simulink model "sampleModel371"  (R2021b)
settings: Solver=VariableStepAuto  StartTime=0.0  StopTime=10.0  RelTol=1e-3
undefined symbols (not defined in the file or in its folder): DiscIntNeverNeededParam, Newton, Raphson
libraries: simulink x16, slpidlib x1
settings Model: Creator=user  LastModifiedBy=user

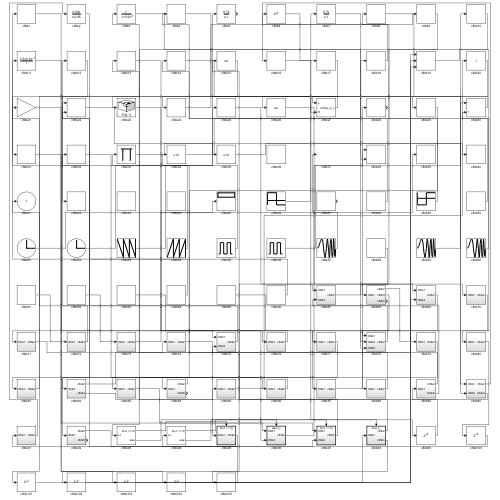
[thumbnail: Simulink's stored preview of the top-level diagram]
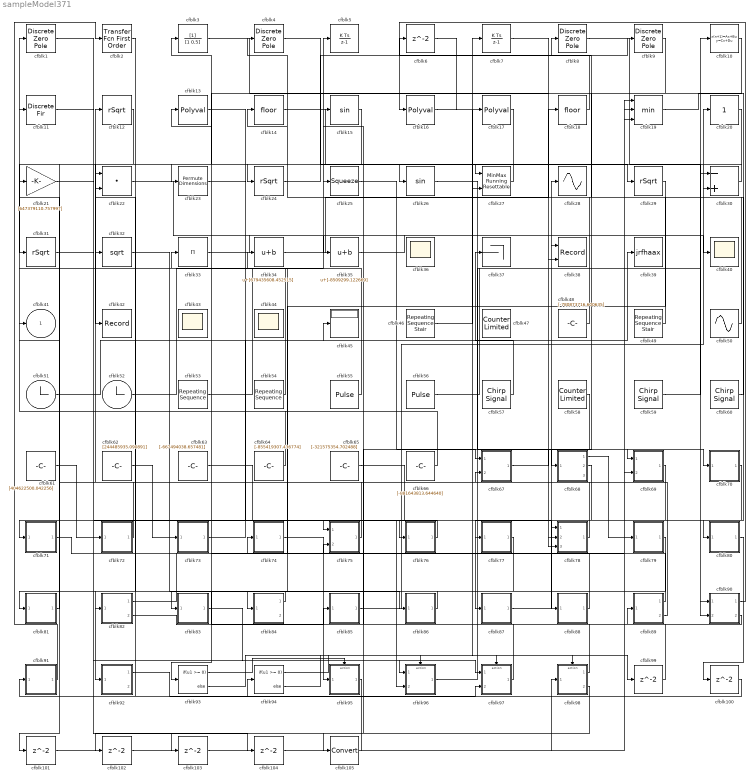
== system sampleModel371 ==
  cfblk{1,4,8..9} (4 alike) : DiscreteZeroPole  Poles=[0 0.5]  Gain=1
  cfblk10 : DiscreteStateSpace
  cfblk{6,99..104} (7 alike) : Delay  SampleTime=1
  cfblk105 : DataTypeConversion
  cfblk11 : DiscreteFir  SampleTime=1
  cfblk{12,24,29,31} (4 alike) : Sqrt  Operator=rSqrt  AlgorithmType=Newton-Raphson  SaturateOnIntegerOverflow=on
  cfblk13 : Polyval  Coefs=[ +2.081618890e-019, -1.441693666e-014, +4.719686976e-010, -8.536869453e-006, +1.621573104e-001, -8.087801117e+001 ]
  cfblk14 : Rounding
  cfblk15 : Trigonometry
  cfblk16 : Polyval  Coefs=[ +2.081618890e-019, -1.441693666e-014, +4.719686976e-010, -8.536869453e-006, +1.621573104e-001, -8.087801117e+001 ]
  cfblk17 : Polyval  Coefs=[ +2.081618890e-019, -1.441693666e-014, +4.719686976e-010, -8.536869453e-006, +1.621573104e-001, -8.087801117e+001 ]
  cfblk18 : Rounding
  cfblk19 : MinMax  Inputs=3
  cfblk2 : simulink/Discrete/Transfer Fcn First Order  PoleZ=0.95  ICPrevOutput=0.0  DoSatur=off
  cfblk20 : simulink/Math Operations/Slider Gain  gain=1  low=0  high=2
  cfblk21 : Gain  Gain=[647379110.757997]
  cfblk22 : DotProduct  InputSameDT=on  OutDataTypeStr=Inherit: Inherit via internal rule
  cfblk23 : PermuteDimensions
  cfblk25 : Squeeze
  cfblk26 : Trigonometry
  cfblk27 : simulink/Math Operations/MinMax Running Resettable  Function=min  vinit=0.0
  cfblk28 : Sin  TimeSource=Use external signal  SampleTime=0
  cfblk3 : DiscreteFilter  SampleTime=1
  cfblk30 : Sum  Inputs=-+
  cfblk32 : Sqrt  SaturateOnIntegerOverflow=on
  cfblk33 : Product  Inputs=*
  cfblk34 : Bias  Bias=[679435608.452515]
  cfblk35 : Bias  Bias=[-8509299.122669]
  cfblk{36,40,43..44} (4 alike) : Scope
      cfblk36 settings: Floating=on
      cfblk43 settings: Floating=on
      cfblk44 settings: Floating=on
  cfblk37 : Terminator
  cfblk38 : Record  FileSettingsInternal="{\"entries\":[{\"content\":{\"excelSettings\":{\"content\":{},\"type\":\"Streamout.ExcelSettings\"}},\"type\":\"Streamout.FileSettingStorage\",\"uuid\":\"9fc04052-8b8e-4725-86d2-7cf5f812b2a1\"}],\"packageUris\":[\"http://schema.mathworks.com/mf0/streamout_blocks/R2020a\"],\"version\":\"1.0\"}"  Layout=[1 1]  SignalsInternal="{\"entries\":[{\"content\":{\"signals\":[{\"content\":{\"blockPath\":[\"sampleModel371/cfblk38\"],\"channel\":[],\"dimensions\":[1],\"domain\":\"sampleModel371/cfblk38\",\"lineColor\":\"#a2142f\",\"plots\":[1],\"port\":1,\"sid\":[\"\"],\"signalID\":15418,\"signalName\":\"cfblk96\"},\"type\":\"RecordBlkView.Signal\",\"uuid\":\"3d61ea52-26a8-4207-9b7d-ce4d298dc0bd\"},{\"content\":{\"blockPath\":[\"sampleModel371/cfblk38\"],\"channel\":[],\"dimensions\":[1],\"domain\":\"sampleModel371/cfblk38\",\"lineColor\":\"#139fff\",\"plots\":[1],\"port\":2,\"sid\":[\"\"],\"signalID\":15422,\"signalName\":\"cfblk3\"},\"type\":\"RecordBlkView.Signal\",\"uuid\":\"41d0d82b-847e-4e7e-9938-72f6bd31de9c\"}]},\"type\":\"RecordBlkView.InputSignals\",\"uuid\":\"d21ca9dd-40f7-4d18-b4d9-355bbf76461b\"}],\"packageUris\":[\"http://schema.mathworks.com/mf0/streamout_blocks/R2020a\"],\"version\":\"1.0\"}"  VisualizationBindings="{\"xyplotplugin\":{\"info\":[{\"series\":[{\"bindingParametersList\":[{\"parameter\":\"X-Axis\",\"signalID\":15418,\"signalName\":\"cfblk96\"},{\"parameter\":\"Y-Axis\",\"signalID\":15422,\"signalName\":\"cfblk3\"}],\"seriesID\":59305}],\"subplotID\":1}]}}"  CompatibilityTag=XY
  cfblk39 : ToWorkspace  VariableName=jrfhaax  SaveFormat=Timeseries  SampleTime=-1
  cfblk42 : Record  FileSettingsInternal="{\"entries\":[{\"content\":{\"excelSettings\":{\"content\":{},\"type\":\"Streamout.ExcelSettings\"}},\"type\":\"Streamout.FileSettingStorage\",\"uuid\":\"b9a56b8f-e8fc-4666-a556-652c0deea9d6\"}],\"packageUris\":[\"http://schema.mathworks.com/mf0/streamout_blocks/R2020a\"],\"version\":\"1.0\"}"  SignalsInternal="{\"entries\":[{\"content\":{\"signals\":[{\"content\":{\"blockPath\":[\"sampleModel371/cfblk42\"],\"channel\":[],\"dimensions\":[1],\"domain\":\"sampleModel371/cfblk42\",\"lineColor\":\"#0072bd\",\"plots\":[1],\"port\":1,\"sid\":[\"\"],\"signalID\":15426,\"signalName\":\"cfblk12\"},\"type\":\"RecordBlkView.Signal\",\"uuid\":\"61be2cdd-bcd1-4740-b751-c89f055e617a\"}]},\"type\":\"RecordBlkView.InputSignals\",\"uuid\":\"9fe64509-3397-4dbe-9be9-cbf438e67b07\"}],\"packageUris\":[\"http://schema.mathworks.com/mf0/streamout_blocks/R2020a\"],\"version\":\"1.0\"}"  VisualizationBindings="{\"sparklinesplugin\":{\"info\":[{\"bindingParametersList\":[],\"subplotID\":1}]}}"
  cfblk45 : Display
  cfblk46 : simulink/Sources/Repeating Sequence Stair  OutValues=[875396539.416185, -474636717.858967]  tsamp=-1  OutMin=[]  OutMax=[]  OutDataTypeStr=double  OutputDataTypeScalingMode=double  OutDataType=fixdt(0,8)  ConRadixGroup=Best Precision: Vector-wise  OutScaling=2^-12
  cfblk47 : simulink/Sources/Counter Limited  uplimit=[503.000000]  tsamp=-1
  cfblk48 : Constant  Value=[-780873716.600635]  SampleTime=1
  cfblk49 : simulink/Sources/Repeating Sequence Stair  OutValues=[-638428813.350056, 591562095.048275]  tsamp=-1  OutMin=[]  OutMax=[]  OutDataTypeStr=double  OutputDataTypeScalingMode=double  OutDataType=fixdt(0,8)  ConRadixGroup=Best Precision: Vector-wise  OutScaling=2^-12
  cfblk5 : DiscreteIntegrator  ICPrevOutput=DiscIntNeverNeededParam  ICPrevScaledInput=DiscIntNeverNeededParam
  cfblk50 : Sin  Amplitude=[814277309.759991]  Bias=[541474944.272401]  SampleTime=0
  cfblk51 : Clock
  cfblk52 : Clock
  cfblk53 : simulink/Sources/Repeating Sequence  rep_seq_t=[0 2]  rep_seq_y=[845598194.254567, 45370993.914203]
  cfblk54 : simulink/Sources/Repeating Sequence  rep_seq_t=[0 2]  rep_seq_y=[-622327897.536918, 514712392.669646]
  cfblk55 : DiscretePulseGenerator  PulseType=Time based  Amplitude=[944860863.611499]  Period=[65183913.372249]  PulseWidth=5  PhaseDelay=[8.000000]
  cfblk56 : DiscretePulseGenerator  PulseType=Time based  Amplitude=[-618955552.202892]  Period=[96517376.948850]  PulseWidth=5  PhaseDelay=[6.000000]
  cfblk57 : simulink/Sources/Chirp Signal  f1=[-190410484.852389]  T=[-195836475.301159]  f2=[603076761.049047]
  cfblk58 : simulink/Sources/Counter Limited  uplimit=[276.000000]  tsamp=-1
  cfblk59 : simulink/Sources/Chirp Signal  f1=[606511793.008932]  T=[320109653.210944]  f2=[959584980.441346]
  cfblk60 : simulink/Sources/Chirp Signal  f1=[-875766691.668898]  T=[126991163.871729]  f2=[-767987395.473026]
  cfblk61 : Constant  Value=[404622500.042256]  SampleTime=1
  cfblk62 : Constant  Value=[244485935.090891]  SampleTime=1
  cfblk63 : Constant  Value=[-667494038.657481]  SampleTime=1
  cfblk64 : Constant  Value=[-855419307.436774]  SampleTime=1
  cfblk65 : Constant  Value=[-321575354.702488]  SampleTime=1
  cfblk66 : Constant  Value=[-881643813.644640]  SampleTime=1
  cfblk67 : Subsystem
  cfblk68 : Subsystem
  cfblk69 : Subsystem
  cfblk7 : DiscreteIntegrator  ICPrevOutput=DiscIntNeverNeededParam  ICPrevScaledInput=DiscIntNeverNeededParam
  cfblk70 : Subsystem
  cfblk71 : Subsystem
  cfblk72 : Subsystem
  cfblk73 : Subsystem
  cfblk74 : Subsystem
  cfblk75 : Subsystem
  cfblk76 : Subsystem
  cfblk77 : Subsystem
  cfblk78 : Subsystem
  cfblk79 : Subsystem
  cfblk80 : Subsystem
  cfblk81 : Subsystem
  cfblk82 : Subsystem
  cfblk83 : Subsystem
  cfblk84 : Subsystem
  cfblk85 : Subsystem
  cfblk86 : Subsystem
  cfblk87 : Subsystem
  cfblk88 : Subsystem
  cfblk89 : Subsystem
  cfblk90 : Subsystem
  cfblk91 : Subsystem
  cfblk92 : Subsystem
  cfblk93 : If  IfExpression=u1 >= 0  SampleTime=1
  cfblk94 : If  IfExpression=u1 >= 0  SampleTime=1
  cfblk95 : Subsystem  TreatAsAtomicUnit=on
  cfblk96 : Subsystem  TreatAsAtomicUnit=on
  cfblk97 : Subsystem  TreatAsAtomicUnit=on
  cfblk98 : Subsystem  TreatAsAtomicUnit=on
  cfblk41 : Outport
  wires:
  cfblk51/1 -> cfblk39/1
  cfblk61/1 -> cfblk72/1(cfblk1)
  cfblk85/1(cfblk2) -> cfblk20/1
  cfblk62/1 -> cfblk73/1(cfblk1)
  cfblk76/1(cfblk2) -> cfblk71/1(cfblk1)
  cfblk87/1(cfblk2) -> cfblk28/1
  cfblk71/1(cfblk2) -> cfblk74/1(cfblk1)
  cfblk96/1(cfblk2) -> cfblk38/1
  cfblk49/1 -> cfblk8/1
  cfblk64/1 -> cfblk1/1
  cfblk29/1 -> cfblk84/1(cfblk1)
  cfblk72/1(cfblk2) -> cfblk12/1
  cfblk52/1 -> cfblk5/1
  cfblk65/1 -> cfblk87/1(cfblk1)
  cfblk35/1 -> cfblk40/1
  cfblk19/1 -> cfblk80/1(cfblk1)
  cfblk81/1(cfblk2) -> cfblk41/1
  cfblk79/1(cfblk2) -> cfblk92/1(cfblk1)
  cfblk12/1 -> cfblk42/1
  cfblk90/1(cfblk2) -> cfblk16/1
  cfblk9/1 -> cfblk68/1(cfblk1)
  cfblk59/1 -> cfblk10/1
  cfblk86/1(cfblk2) -> cfblk81/1(cfblk1)
  cfblk30/1 -> cfblk26/1
  cfblk26/1 -> cfblk70/1(cfblk1)
  cfblk83/1(cfblk2) -> cfblk96/1(cfblk1)
  cfblk74/1(cfblk2) -> cfblk95/1(cfblk1)
  cfblk56/1 -> cfblk30/1
  cfblk55/1 -> cfblk11/1
  cfblk4/1 -> cfblk29/1
  cfblk97/1(cfblk2) -> cfblk13/1
  cfblk54/1 -> cfblk3/1
  cfblk60/1 -> cfblk30/2
  cfblk20/1 -> cfblk31/1
  cfblk68/1(cfblk2) -> cfblk79/1(cfblk1)
  cfblk27/1 -> cfblk24/1
  cfblk53/1 -> cfblk25/1
  cfblk73/1(cfblk2) -> cfblk45/1
  cfblk48/1 -> cfblk14/1
  cfblk34/1 -> cfblk18/1
  cfblk75/1(cfblk2) -> cfblk22/1
  cfblk8/1 -> cfblk90/1(cfblk1)
  cfblk2/1 -> cfblk82/1(cfblk1)
  cfblk6/1 -> cfblk17/1
  cfblk70/1(cfblk2) -> cfblk77/1(cfblk1)
  cfblk24/1 -> cfblk9/1
  cfblk89/1(cfblk2) -> cfblk33/1
  cfblk22/1 -> cfblk90/2(cfblk3)
  cfblk17/1 -> cfblk27/1
  cfblk95/1(cfblk2) -> cfblk91/1(cfblk1)
  cfblk25/1 -> cfblk67/1(cfblk1)
  cfblk90/2(cfblk4) -> cfblk89/1(cfblk1)
  cfblk84/1(cfblk2) -> cfblk83/1(cfblk1)
  cfblk69/1(cfblk2) -> cfblk88/1(cfblk1)
  cfblk10/1 -> cfblk23/1
  cfblk77/1(cfblk2) -> cfblk93/1
  cfblk14/1 -> cfblk27/2
  cfblk57/1 -> cfblk37/1
  cfblk82/1(cfblk2) -> cfblk19/1
  cfblk3/1 -> cfblk38/2
  cfblk13/1 -> cfblk76/1(cfblk1)
  cfblk78/1(cfblk2) -> cfblk21/1
  cfblk18/1 -> cfblk6/1
  cfblk50/1 -> cfblk4/1
  cfblk33/1 -> cfblk35/1
  cfblk46/1 -> cfblk7/1
  cfblk32/1 -> cfblk86/1(cfblk1)
  cfblk23/1 -> cfblk78/1(cfblk1)
  cfblk11/1 -> cfblk97/1(cfblk1)
  cfblk82/2(cfblk4) -> cfblk85/1(cfblk1)
  cfblk66/1 -> cfblk32/1
  cfblk67/1(cfblk2) -> cfblk69/1(cfblk1)
  cfblk88/1(cfblk2) -> cfblk34/1
  cfblk98/1(cfblk2) -> cfblk15/1
  cfblk91/1(cfblk2) -> cfblk2/1
  cfblk7/1 -> cfblk78/2(cfblk4)
  cfblk89/2(cfblk5) -> cfblk67/2(cfblk4)
  cfblk68/2(cfblk3) -> cfblk78/3(cfblk5)
  cfblk1/1 -> cfblk75/1(cfblk1)
  cfblk92/1(cfblk2) -> cfblk97/2(cfblk4)
  cfblk63/1 -> cfblk96/2(cfblk3)
  cfblk93/1 -> cfblk95/Action
  cfblk93/2 -> cfblk96/Action
  cfblk94/1 -> cfblk97/Action
  cfblk94/2 -> cfblk98/Action
  cfblk16/1 -> cfblk99/1
  cfblk99/1 -> cfblk75/2(cfblk4)
  cfblk80/1(cfblk2) -> cfblk100/1
  cfblk100/1 -> cfblk94/1
  cfblk15/1 -> cfblk101/1
  cfblk101/1 -> cfblk19/2
  cfblk98/2(cfblk4) -> cfblk102/1
  cfblk102/1 -> cfblk19/3
  cfblk31/1 -> cfblk103/1
  cfblk103/1 -> cfblk98/1(cfblk1)
  cfblk21/1 -> cfblk104/1
  cfblk104/1 -> cfblk69/2(cfblk4)
  cfblk58/1 -> cfblk105/1
  cfblk105/1 -> cfblk22/2

== system sampleModel371/cfblk67 ==
  cfblk1 : Inport
  cfblk4 : Inport  Port=2
  cfblk3 : UnaryMinus
  cfblk2 : Outport
  wires:
  cfblk1/1 -> cfblk2/1
  cfblk4/1 -> cfblk3/1

== system sampleModel371/cfblk68 ==
  cfblk1 : Inport
  cfblk2 : Outport
  cfblk3 : Outport  Port=2
  cfblk4 : Outport  Port=3
  wires:
  cfblk1/1 -> cfblk2/1, cfblk4/1, cfblk3/1

== system sampleModel371/cfblk69 ==
  cfblk1 : Inport
  cfblk4 : Inport  Port=2
  cfblk3 : UnitDelay  HasFrameUpgradeWarning=on
  cfblk2 : Outport
  wires:
  cfblk1/1 -> cfblk3/1
  cfblk4/1 -> cfblk2/1

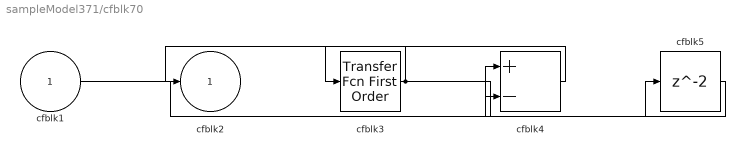
== system sampleModel371/cfblk70 ==
  cfblk1 : Inport
  cfblk3 : simulink/Discrete/Transfer Fcn First Order  PoleZ=0.95  ICPrevOutput=0.0  DoSatur=off
  cfblk4 : Sum  Inputs=+-
  cfblk5 : Delay  SampleTime=1
  cfblk2 : Outport
  wires:
  cfblk4/1 -> cfblk3/1
  cfblk1/1 -> cfblk4/1
  cfblk3/1 -> cfblk2/1, cfblk5/1
  cfblk5/1 -> cfblk4/2

== system sampleModel371/cfblk71 ==
  cfblk1 : Inport
  cfblk3 : Bias  Bias=[-84234568.699611]
  cfblk2 : Outport
  wires:
  cfblk1/1 -> cfblk3/1
  cfblk3/1 -> cfblk2/1

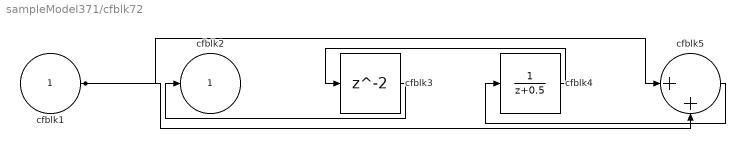
== system sampleModel371/cfblk72 ==
  cfblk1 : Inport
  cfblk3 : Delay  SampleTime=1
  cfblk4 : DiscreteTransferFcn  SampleTime=1
  cfblk5 : Sum  Inputs=|++
  cfblk2 : Outport
  wires:
  cfblk4/1 -> cfblk3/1
  cfblk3/1 -> cfblk2/1
  cfblk1/1 -> cfblk5/1, cfblk5/2
  cfblk5/1 -> cfblk4/1

== system sampleModel371/cfblk73 ==
  cfblk1 : Inport
  cfblk3 : DiscreteIntegrator  ICPrevOutput=DiscIntNeverNeededParam  ICPrevScaledInput=DiscIntNeverNeededParam
  cfblk4 : Constant  Value=[552070176.584629]  SampleTime=1
  cfblk2 : Outport
  wires:
  cfblk1/1 -> cfblk3/1
  cfblk3/1 -> cfblk2/1

== system sampleModel371/cfblk74 ==
  cfblk1 : Inport
  cfblk3 : DiscreteFir  SampleTime=1
  cfblk2 : Outport
  wires:
  cfblk1/1 -> cfblk3/1
  cfblk3/1 -> cfblk2/1

== system sampleModel371/cfblk75 ==
  cfblk1 : Inport
  cfblk4 : Inport  Port=2
  cfblk3 : DiscreteIntegrator  ICPrevOutput=DiscIntNeverNeededParam  ICPrevScaledInput=DiscIntNeverNeededParam
  cfblk2 : Outport
  wires:
  cfblk1/1 -> cfblk2/1
  cfblk4/1 -> cfblk3/1

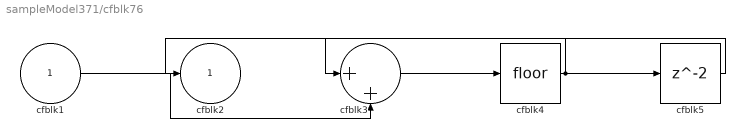
== system sampleModel371/cfblk76 ==
  cfblk1 : Inport
  cfblk3 : Sum  Inputs=|++
  cfblk4 : Rounding
  cfblk5 : Delay  SampleTime=1
  cfblk2 : Outport
  wires:
  cfblk3/1 -> cfblk4/1
  cfblk4/1 -> cfblk2/1, cfblk5/1
  cfblk1/1 -> cfblk3/2
  cfblk5/1 -> cfblk3/1

== system sampleModel371/cfblk77 ==
  cfblk1 : Inport
  cfblk3 : UnitDelay  HasFrameUpgradeWarning=on
  cfblk2 : Outport
  wires:
  cfblk3/1 -> cfblk2/1
  cfblk1/1 -> cfblk3/1

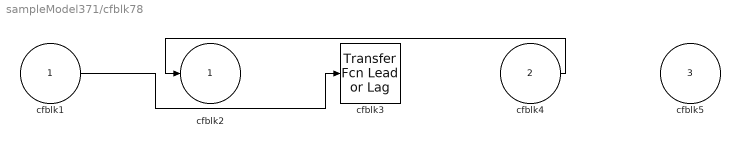
== system sampleModel371/cfblk78 ==
  cfblk1 : Inport
  cfblk4 : Inport  Port=2
  cfblk5 : Inport  Port=3
  cfblk3 : simulink/Discrete/Transfer Fcn Lead or Lag  PoleZ=0.95  ZeroZ=0.75  ICPrevOutput=0.0  ICPrevInput=0.0  DoSatur=off
      settings: SourceProductBaseCode=SL
  cfblk2 : Outport
  wires:
  cfblk4/1 -> cfblk2/1
  cfblk1/1 -> cfblk3/1

== system sampleModel371/cfblk79 ==
  cfblk1 : Inport
  cfblk3 : Constant  Value=[1854064.119149]  SampleTime=1
  cfblk2 : Outport
  wires:
  cfblk1/1 -> cfblk2/1

== system sampleModel371/cfblk80 ==
  cfblk1 : Inport
  cfblk3 : simulink/Discrete/Transfer Fcn Lead or Lag  PoleZ=0.95  ZeroZ=0.75  ICPrevOutput=0.0  ICPrevInput=0.0  DoSatur=off
      settings: SourceProductBaseCode=SL
  cfblk4 : Constant  Value=[-147275204.344261]  SampleTime=1
  cfblk2 : Outport
  wires:
  cfblk4/1 -> cfblk3/1
  cfblk1/1 -> cfblk2/1

== system sampleModel371/cfblk81 ==
  cfblk1 : Inport
  cfblk3 : Bias  Bias=[-489487541.213610]
  cfblk4 : Constant  Value=[323034840.846709]  SampleTime=1
  cfblk2 : Outport
  wires:
  cfblk1/1 -> cfblk3/1
  cfblk3/1 -> cfblk2/1

== system sampleModel371/cfblk82 ==
  cfblk1 : Inport
  cfblk3 : Delay  DelayLengthSource=Input port  SampleTime=1
      settings: InputPortMap=u0,p1
  cfblk2 : Outport
  cfblk4 : Outport  Port=2
  wires:
  cfblk1/1 -> cfblk4/1, cfblk3/1, cfblk3/2
  cfblk3/1 -> cfblk2/1

== system sampleModel371/cfblk83 ==
  cfblk1 : Inport
  cfblk3 : DiscreteTransferFcn  SampleTime=1
  cfblk2 : Outport
  wires:
  cfblk1/1 -> cfblk3/1
  cfblk3/1 -> cfblk2/1

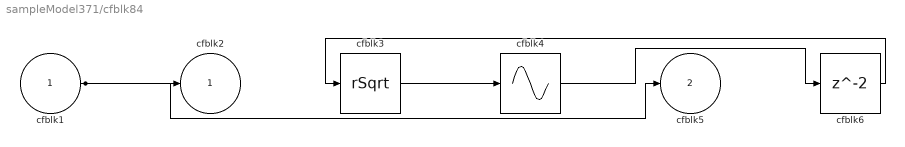
== system sampleModel371/cfblk84 ==
  cfblk1 : Inport
  cfblk3 : Sqrt  Operator=rSqrt  AlgorithmType=Newton-Raphson  SaturateOnIntegerOverflow=on
  cfblk4 : Sin  TimeSource=Use external signal  SampleTime=0
  cfblk6 : Delay  SampleTime=1
  cfblk2 : Outport
  cfblk5 : Outport  Port=2
  wires:
  cfblk3/1 -> cfblk4/1
  cfblk1/1 -> cfblk5/1, cfblk2/1
  cfblk4/1 -> cfblk6/1
  cfblk6/1 -> cfblk3/1

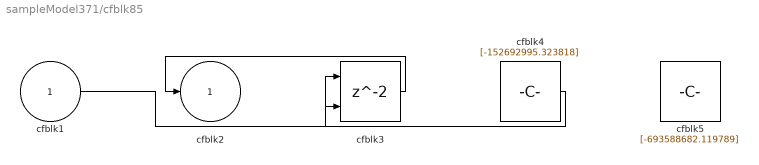
== system sampleModel371/cfblk85 ==
  cfblk1 : Inport
  cfblk3 : Delay  ShowEnablePort=on  SampleTime=1
      settings: InputPortMap=u0,e6
  cfblk4 : Constant  Value=[-152692995.323818]  SampleTime=1
  cfblk5 : Constant  Value=[-693588682.119789]  SampleTime=1
  cfblk2 : Outport
  wires:
  cfblk3/1 -> cfblk2/1
  cfblk1/1 -> cfblk3/1
  cfblk4/1 -> cfblk3/2

== system sampleModel371/cfblk86 ==
  cfblk1 : Inport
  cfblk3 : Rounding
  cfblk2 : Outport
  wires:
  cfblk1/1 -> cfblk3/1
  cfblk3/1 -> cfblk2/1

== system sampleModel371/cfblk87 ==
  cfblk1 : Inport
  cfblk3 : Reshape
  cfblk2 : Outport
  wires:
  cfblk1/1 -> cfblk2/1, cfblk3/1

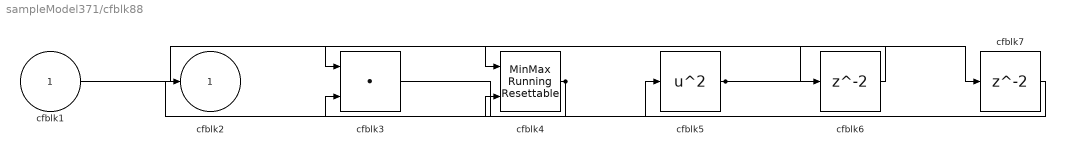
== system sampleModel371/cfblk88 ==
  cfblk1 : Inport
  cfblk3 : DotProduct  InputSameDT=on  OutDataTypeStr=Inherit: Inherit via internal rule
  cfblk4 : simulink/Math Operations/MinMax Running Resettable  Function=min  vinit=0.0
  cfblk5 : Math  Operator=square  SaturateOnIntegerOverflow=on
  cfblk6 : Delay  SampleTime=1
  cfblk7 : Delay  SampleTime=1
  cfblk2 : Outport
  wires:
  cfblk1/1 -> cfblk4/1
  cfblk4/1 -> cfblk2/1, cfblk3/2
  cfblk5/1 -> cfblk6/1, cfblk7/1
  cfblk3/1 -> cfblk5/1
  cfblk6/1 -> cfblk3/1
  cfblk7/1 -> cfblk4/2

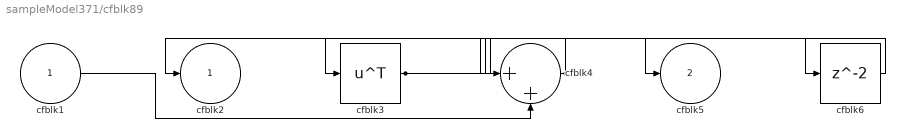
== system sampleModel371/cfblk89 ==
  cfblk1 : Inport
  cfblk3 : Math  Operator=transpose  SaturateOnIntegerOverflow=on
  cfblk4 : Sum  Inputs=|++
  cfblk6 : Delay  SampleTime=1
  cfblk2 : Outport
  cfblk5 : Outport  Port=2
  wires:
  cfblk3/1 -> cfblk5/1, cfblk6/1
  cfblk4/1 -> cfblk2/1, cfblk3/1
  cfblk1/1 -> cfblk4/2
  cfblk6/1 -> cfblk4/1

== system sampleModel371/cfblk90 ==
  cfblk1 : Inport
  cfblk3 : Inport  Port=2
  cfblk2 : Outport
  cfblk4 : Outport  Port=2
  wires:
  cfblk1/1 -> cfblk2/1
  cfblk3/1 -> cfblk4/1

== system sampleModel371/cfblk91 ==
  cfblk1 : Inport
  cfblk3 : Sin  TimeSource=Use external signal  SampleTime=0
  cfblk4 : Constant  Value=[-497411138.577247]  SampleTime=1
  cfblk2 : Outport
  wires:
  cfblk3/1 -> cfblk2/1
  cfblk4/1 -> cfblk3/1

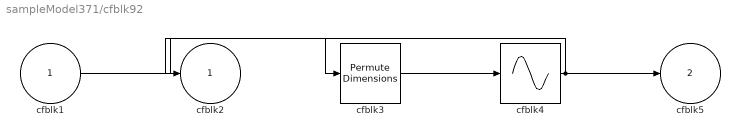
== system sampleModel371/cfblk92 ==
  cfblk1 : Inport
  cfblk3 : PermuteDimensions
  cfblk4 : Sin  TimeSource=Use external signal  SampleTime=0
  cfblk2 : Outport
  cfblk5 : Outport  Port=2
  wires:
  cfblk1/1 -> cfblk3/1
  cfblk3/1 -> cfblk4/1
  cfblk4/1 -> cfblk5/1, cfblk2/1

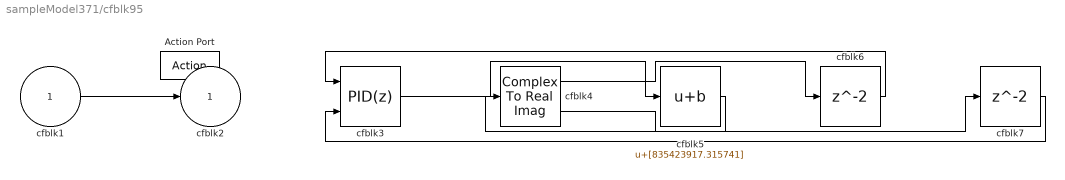
== system sampleModel371/cfblk95 ==
  cfblk1 : Inport
  Action Port : ActionPort  ActionPortLabel=if(u1 >= 0)
  cfblk3 : slpidlib/PID Controller (2DOF)  Controller=PID  Form=Parallel  TimeDomain=Discrete-time  UseExternalTs=off  SampleTime=-1  IntegratorMethod=Forward Euler  FilterMethod=Forward Euler  ControllerParametersSource=internal  P=1  I=1  D=0  UseFilter=on  N=100  b=1  c=1  TunerSelectOption=Transfer Function Based (PID Tuner App)  InitialConditionSource=internal  InitialConditionForIntegrator=0  InitialConditionForFilter=0  DifferentiatorICPrevScaledInput=0  ExternalReset=none  TrackingMode=off  Kt=1  LimitOutput=off  SatLimitsSource=internal  UpperSaturationLimit=inf  LowerSaturationLimit=-inf  LinearizeAsGain=off  AntiWindupMode=none  Kb=1  POutMin=[]  POutMax=[]  IOutMin=[]  IOutMax=[]  DOutMin=[]  DOutMax=[]  NOutMin=[]  NOutMax=[]  bOutMin=[]  bOutMax=[]  cOutMin=[]  cOutMax=[]  SumOutMin=[]  SumOutMax=[]  SaturationOutMin=[]  SaturationOutMax=[]  PParamMin=[]  PParamMax=[]  IParamMin=[]  IParamMax=[]  DParamMin=[]  DParamMax=[]  NParamMin=[]  NParamMax=[]  bParamMin=[]  bParamMax=[]  cParamMin=[]  cParamMax=[]  KbParamMin=[]  KbParamMax=[]  KtParamMin=[]  KtParamMax=[]  KbOutMin=[]  KbOutMax=[]  KtOutMin=[]  KtOutMax=[]  IntegratorOutMin=[]  IntegratorOutMax=[]  FilterOutMin=[]  FilterOutMax=[]  SumI1OutMin=[]  SumI1OutMax=[]  SumI2OutMin=[]  SumI2OutMax=[]  SumI3OutMin=[]  SumI3OutMax=[]  SumI4OutMin=[]  SumI4OutMax=[]  SumDOutMin=[]  SumDOutMax=[]  Sum1OutMin=[]  Sum1OutMax=[]  Sum2OutMin=[]  Sum2OutMax=[]  Sum3OutMin=[]  Sum3OutMax=[]  DifferentiatorOutMin=[]  DifferentiatorOutMax=[]  FilterDiffOutCoefMin=[]  FilterDiffOutCoefMax=[]  ReciprocalOutMin=[]  ReciprocalOutMax=[]  SumDenOutMin=[]  SumDenOutMax=[]  SumNumOutMin=[]  SumNumOutMax=[]  DivideOutMin=[]  DivideOutMax=[]  UdiffTsProdOutMin=[]  UdiffTsProdOutMax=[]  NTsProdOutMin=[]  NTsProdOutMax=[]  UintegralTsProdOutMin=[]  UintegralTsProdOutMax=[]  UngainTsProdOutMin=[]  UngainTsProdOutMax=[]  IntegratorContinuousStateAttributes=''  IntegratorStateMustResolveToSignalObject=off  IntegratorRTWStateStorageClass=Auto  FilterContinuousStateAttributes=''  FilterStateMustResolveToSignalObject=off  FilterRTWStateStorageClass=Auto  ParallelPVariant=InternalParameters  IdealPVariant=Disabled  IVariant=InternalParameters  DVariant=InternalParameters  bVariant=InternalParameters  cVariant=InternalParameters  IntegratorVariant=Discrete  SatVariant=Disabled  AWVariant=Passthrough  PCopyVariant=Disabled  TRVariant=Disabled  FdbkBlocksVariant=Forward  IdealPFdbkVariant=Disabled  SatFdbkVariant=Disabled  DerivativeFilterVariant=ForwardEulerFilter  NVariant=InternalParameters  NCopyVariant=Disabled  FilterICVariant=InternalICsFilter  IntegratorICVariant=InternalICs  ExternalResetVariant=Disabled  TRSumVariant=Passthrough  SumFdbkVariant=Disabled  SumVariant=Sum_PID  TsampFilterVariant=InternalTs  TsampNgainVariant=Passthrough  TsampIntegralVariant=Passthrough  ExternalSaturationOutDataTypeStr=Inherit: Same as second input
      settings: SourceProductBaseCode=SL
  cfblk4 : ComplexToRealImag
  cfblk5 : Bias  Bias=[835423917.315741]
  cfblk6 : Delay
  cfblk7 : Delay
  cfblk2 : Outport
  wires:
  cfblk3/1 -> cfblk5/1
  cfblk5/1 -> cfblk4/1
  cfblk1/1 -> cfblk2/1
  cfblk4/1 -> cfblk6/1
  cfblk6/1 -> cfblk3/1
  cfblk4/2 -> cfblk7/1
  cfblk7/1 -> cfblk3/2

== system sampleModel371/cfblk96 ==
  cfblk1 : Inport
  cfblk3 : Inport  Port=2
  Action Port : ActionPort  ActionPortLabel=else
  cfblk2 : Outport
  wires:
  cfblk1/1 -> cfblk2/1

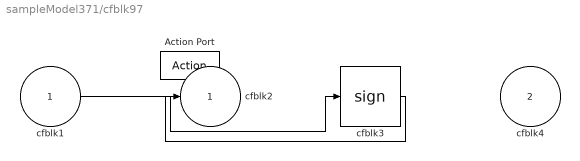
== system sampleModel371/cfblk97 ==
  cfblk1 : Inport
  cfblk4 : Inport  Port=2
  Action Port : ActionPort  ActionPortLabel=if(u1 >= 0)
  cfblk3 : Signum
  cfblk2 : Outport
  wires:
  cfblk1/1 -> cfblk3/1
  cfblk3/1 -> cfblk2/1

== system sampleModel371/cfblk98 ==
  cfblk1 : Inport
  Action Port : ActionPort  ActionPortLabel=else
  cfblk3 : Delay
  cfblk2 : Outport
  cfblk4 : Outport  Port=2
  wires:
  cfblk1/1 -> cfblk2/1, cfblk3/1
  cfblk3/1 -> cfblk4/1
